simulink model "single_link"  (R2023b)
settings: Solver=VariableStepAuto  StartTime=0.0  StopTime=100  RelTol=1e-3
undefined symbols (not defined in the file): X, Y, Z
libraries: sm_lib x10, nesl_utility x3
settings Model: Creator=Admin  LastModifiedBy=gughan
settings ModelReferenceCC: EnableRefExpFcnMdlSchedulingChecks=on

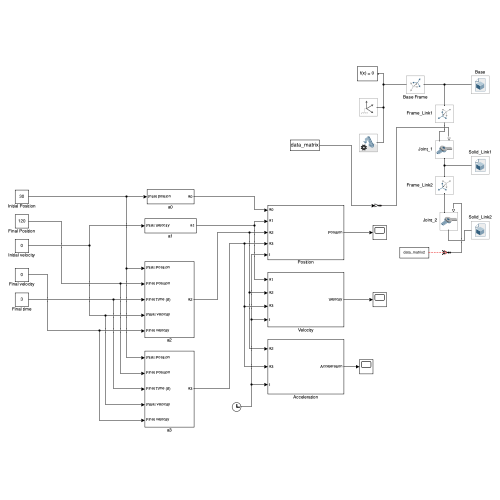
[thumbnail: Simulink's stored preview of the top-level diagram]
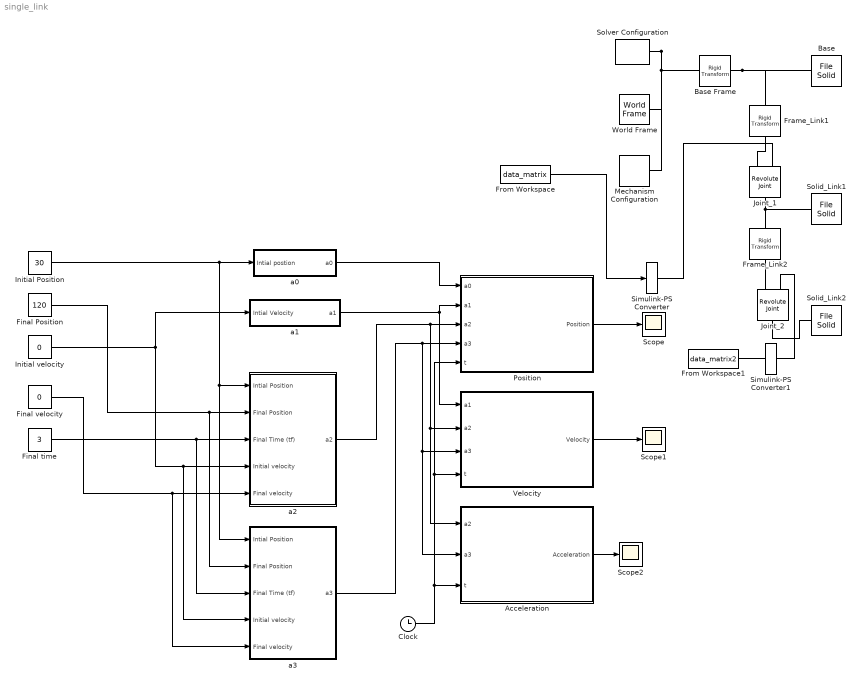
== system single_link ==
  Acceleration : Subsystem
  Base : sm_lib/Body Elements/File Solid  ExtGeomFileName=/Users/gughan/Documents/VIT VELLORE STUFFS/TP/base1.STEP  UnitType=FromFile  ExtGeomFileUnits=m  StepReaderType=HEX  ExportConvexHullGeometry=off  InertiaType=CalculateFromGeometry  Mass=1  MassUnits=kg  CenterOfMass=[0 0 0]  CenterOfMassUnits=m  MomentsOfInertia=[1 1 1]  MomentsOfInertiaUnits=kg*m^2  ProductsOfInertia=[0 0 0]  ProductsOfInertiaUnits=kg*m^2  BasedOnType=Density  Density=1000  DensityUnits=kg/m^3  DoExposeReferenceFrame=on  SerializedFrames=<Frames/>  GraphicType=FromGeometry  MarkerShape=Sphere  MarkerSize=10  GraphicVisPropType=SimpleVisualProperties  GraphicDiffuseColor=[0.5 0.5 0.5]  GraphicSpecularColor=[0.5 0.5 0.5 1.0]  GraphicAmbientColor=[0.15 0.15 0.15 1.0]  GraphicEmissiveColor=[0.0 0.0 0.0 1.0]  GraphicShininess=75  GraphicOpacity=1.0
  Base Frame : sm_lib/Frames and Transforms/Rigid Transform  TranslationMethod=Cartesian  TranslationStandardOffset=0  TranslationStandardOffsetUnits=m  TranslationStandardAxis=+Z  TranslationCartesianOffset=[0 0 0]  TranslationCartesianOffsetUnits=m  TranslationROffset=0  TranslationROffsetUnits=m  TranslationZOffset=0  TranslationZOffsetUnits=m  TranslationThetaOffset=0  TranslationThetaOffsetUnits=deg  RotationMethod=None  RotationAngleUnits=deg  RotationStandardAxis=+X  RotationAngle=90  RotationArbitraryAxis=[0 0 1]  FollAlignAxisA=+X  BaseAlignAxisA=+Y  FollAlignAxisB=+Y  BaseAlignAxisB=+Z  RotationSequenceAxes=FollowerAxes  RotationSequence=XYX  RotationSequenceAngles=[0 0 0]  RotationSequenceAnglesUnits=deg  RotationMatrix=[1 0 0; 0 1 0; 0 0 1]  Quaternion=[1 0 0 0]
  Clock : Clock
      settings: Decimation=3
  Final Position : Constant  Value=120
  Final time : Constant  Value=3
  Final velocity : Constant  Value=0
  Frame_Link1 : sm_lib/Frames and Transforms/Rigid Transform  TranslationMethod=Cartesian  TranslationStandardOffset=0  TranslationStandardOffsetUnits=mm  TranslationStandardAxis=+Z  TranslationCartesianOffset=[0 0 15]  TranslationCartesianOffsetUnits=mm  TranslationROffset=0  TranslationROffsetUnits=m  TranslationZOffset=0  TranslationZOffsetUnits=m  TranslationThetaOffset=0  TranslationThetaOffsetUnits=deg  RotationMethod=None  RotationAngleUnits=deg  RotationStandardAxis=+X  RotationAngle=90  RotationArbitraryAxis=[0 0 1]  FollAlignAxisA=+X  BaseAlignAxisA=+Y  FollAlignAxisB=+Y  BaseAlignAxisB=+Z  RotationSequenceAxes=FollowerAxes  RotationSequence=XYX  RotationSequenceAngles=[0 0 0]  RotationSequenceAnglesUnits=deg  RotationMatrix=[1 0 0; 0 1 0; 0 0 1]  Quaternion=[1 0 0 0]
  Frame_Link2 : sm_lib/Frames and Transforms/Rigid Transform  TranslationMethod=Cartesian  TranslationStandardOffset=0  TranslationStandardOffsetUnits=mm  TranslationStandardAxis=+Z  TranslationCartesianOffset=[200 0 10]  TranslationCartesianOffsetUnits=mm  TranslationROffset=0  TranslationROffsetUnits=m  TranslationZOffset=0  TranslationZOffsetUnits=m  TranslationThetaOffset=0  TranslationThetaOffsetUnits=deg  RotationMethod=None  RotationAngleUnits=deg  RotationStandardAxis=+Z  RotationAngle=0.0  RotationArbitraryAxis=[0 0 1]  FollAlignAxisA=+X  BaseAlignAxisA=+Y  FollAlignAxisB=+Y  BaseAlignAxisB=+Z  RotationSequenceAxes=FollowerAxes  RotationSequence=XYX  RotationSequenceAngles=[0 0 0]  RotationSequenceAnglesUnits=deg  RotationMatrix=[1 0 0; 0 1 0; 0 0 1]  Quaternion=[1 0 0 0]
  From Workspace : FromWorkspace  VariableName=data_matrix
  From Workspace1 : FromWorkspace  VariableName=data_matrix2
  Initial Position : Constant  Value=30
  Initial velocity : Constant  Value=0
  Joint_1 : sm_lib/Joints/Revolute Joint  JointMode=Normal  SenseConstraintForce=off  SenseConstraintForceX=off  SenseConstraintForceY=off  SenseConstraintForceZ=off  SenseConstraintTorque=off  SenseConstraintTorqueX=off  SenseConstraintTorqueY=off  SenseConstraintTorqueZ=off  SenseTotalForce=off  SenseTotalForceX=off  SenseTotalForceY=off  SenseTotalForceZ=off  SenseTotalTorque=off  SenseTotalTorqueX=off  SenseTotalTorqueY=off  SenseTotalTorqueZ=off  CompositeWrenchDir=FollowerOnBase  CompositeWrenchFrame=BaseFrame  EquilibriumPosition=0  EquilibriumPositionUnits=deg  SpringStiffness=0  SpringStiffnessUnits=N*m/deg  DampingCoefficient=0  DampingCoefficientUnits=N*m/(deg/s)  TorqueActuationMode=ComputedTorque  MotionActuationMode=InputMotion  SensePosition=off  SenseVelocity=off  SenseAcceleration=off  SenseTorqueForce=off  SenseLowerLimitTorqueForce=off  SenseUpperLimitTorqueForce=off  LowerLimitSpecify=off  LowerLimitBound=-90  LowerLimitBoundUnits=deg  LowerLimitStiffness=1e4  LowerLimitStiffnessUnits=N*m/deg  LowerLimitDamping=10  LowerLimitDampingUnits=N*m/(deg/s)  LowerLimitTransitionRegionWidth=0.1  LowerLimitTransitionRegionWidthUnits=deg  UpperLimitSpecify=off  UpperLimitBound=90  UpperLimitBoundUnits=deg  UpperLimitStiffness=1e4  UpperLimitStiffnessUnits=N*m/deg  UpperLimitDamping=10  UpperLimitDampingUnits=N*m/(deg/s)  UpperLimitTransitionRegionWidth=0.1  UpperLimitTransitionRegionWidthUnits=deg  PositionTargetSpecify=off  PositionTargetPriority=High  PositionTargetValue=0  PositionTargetValueUnits=deg  VelocityTargetSpecify=off  VelocityTargetPriority=High  VelocityTargetValue=0  VelocityTargetValueUnits=deg/s
  Joint_2 : sm_lib/Joints/Revolute Joint  JointMode=Normal  SenseConstraintForce=off  SenseConstraintForceX=off  SenseConstraintForceY=off  SenseConstraintForceZ=off  SenseConstraintTorque=off  SenseConstraintTorqueX=off  SenseConstraintTorqueY=off  SenseConstraintTorqueZ=off  SenseTotalForce=off  SenseTotalForceX=off  SenseTotalForceY=off  SenseTotalForceZ=off  SenseTotalTorque=off  SenseTotalTorqueX=off  SenseTotalTorqueY=off  SenseTotalTorqueZ=off  CompositeWrenchDir=FollowerOnBase  CompositeWrenchFrame=BaseFrame  EquilibriumPosition=0  EquilibriumPositionUnits=deg  SpringStiffness=0  SpringStiffnessUnits=N*m/deg  DampingCoefficient=0  DampingCoefficientUnits=N*m/(deg/s)  TorqueActuationMode=ComputedTorque  MotionActuationMode=InputMotion  SensePosition=off  SenseVelocity=off  SenseAcceleration=off  SenseTorqueForce=off  SenseLowerLimitTorqueForce=off  SenseUpperLimitTorqueForce=off  LowerLimitSpecify=off  LowerLimitBound=-90  LowerLimitBoundUnits=deg  LowerLimitStiffness=1e4  LowerLimitStiffnessUnits=N*m/deg  LowerLimitDamping=10  LowerLimitDampingUnits=N*m/(deg/s)  LowerLimitTransitionRegionWidth=0.1  LowerLimitTransitionRegionWidthUnits=deg  UpperLimitSpecify=off  UpperLimitBound=90  UpperLimitBoundUnits=deg  UpperLimitStiffness=1e4  UpperLimitStiffnessUnits=N*m/deg  UpperLimitDamping=10  UpperLimitDampingUnits=N*m/(deg/s)  UpperLimitTransitionRegionWidth=0.1  UpperLimitTransitionRegionWidthUnits=deg  PositionTargetSpecify=off  PositionTargetPriority=High  PositionTargetValue=0  PositionTargetValueUnits=deg  VelocityTargetSpecify=off  VelocityTargetPriority=High  VelocityTargetValue=0  VelocityTargetValueUnits=deg/s
  Mechanism Configuration : sm_lib/Utilities/Mechanism Configuration  UniformGravity=Constant  GravityVector=[0 0 -9.80665]  GravityVectorUnits=m/s^2  LinearizationDelta=0.001  JointModeTransitionNonlinearIterations=2
  Position : Subsystem
  Scope : Scope
  Scope1 : Scope
  Scope2 : Scope
  Simulink-PS Converter : nesl_utility/Simulink-PS Converter  PhysicalDomain=network_engine_domain  SubClassName=ps_input  LeftPortType=input  RightPortType=output  PseudoPeriodic=off  Frequencies=[]  NoiseDistribution=none  NoiseParameters=[]  Unit=deg  AffineConversion=off  FilteringAndDerivatives=filter  SimscapeFilterOrder=2  InputFilterTimeConstant=.01  UdotUserProvided=0
  Simulink-PS Converter1 : nesl_utility/Simulink-PS Converter  PhysicalDomain=network_engine_domain  SubClassName=ps_input  LeftPortType=input  RightPortType=output  PseudoPeriodic=off  Frequencies=[]  NoiseDistribution=none  NoiseParameters=[]  Unit=deg  AffineConversion=off  FilteringAndDerivatives=filter  SimscapeFilterOrder=2  InputFilterTimeConstant=.01  UdotUserProvided=0
  Solid_Link1 : sm_lib/Body Elements/File Solid  ExtGeomFileName=/Users/gughan/Documents/VIT VELLORE STUFFS/TP/link1.STEP  UnitType=FromFile  ExtGeomFileUnits=m  StepReaderType=HEX  ExportConvexHullGeometry=off  InertiaType=CalculateFromGeometry  Mass=1  MassUnits=kg  CenterOfMass=[0 0 0]  CenterOfMassUnits=m  MomentsOfInertia=[1 1 1]  MomentsOfInertiaUnits=kg*m^2  ProductsOfInertia=[0 0 0]  ProductsOfInertiaUnits=kg*m^2  BasedOnType=Density  Density=1000  DensityUnits=kg/m^3  DoExposeReferenceFrame=on  SerializedFrames=<Frames/>  GraphicType=FromGeometry  MarkerShape=Sphere  MarkerSize=10  GraphicVisPropType=SimpleVisualProperties  GraphicDiffuseColor=[0.5 0.5 0.5]  GraphicSpecularColor=[0.5 0.5 0.5 1.0]  GraphicAmbientColor=[0.15 0.15 0.15 1.0]  GraphicEmissiveColor=[0.0 0.0 0.0 1.0]  GraphicShininess=75  GraphicOpacity=1.0
  Solid_Link2 : sm_lib/Body Elements/File Solid  ExtGeomFileName=/Users/gughan/Documents/VIT VELLORE STUFFS/TP/link1.STEP  UnitType=FromFile  ExtGeomFileUnits=m  StepReaderType=HEX  ExportConvexHullGeometry=off  InertiaType=CalculateFromGeometry  Mass=1  MassUnits=kg  CenterOfMass=[0 0 0]  CenterOfMassUnits=m  MomentsOfInertia=[1 1 1]  MomentsOfInertiaUnits=kg*m^2  ProductsOfInertia=[0 0 0]  ProductsOfInertiaUnits=kg*m^2  BasedOnType=Density  Density=1000  DensityUnits=kg/m^3  DoExposeReferenceFrame=on  SerializedFrames=<Frames/>  GraphicType=FromGeometry  MarkerShape=Sphere  MarkerSize=10  GraphicVisPropType=SimpleVisualProperties  GraphicDiffuseColor=[0.5 0.5 0.5]  GraphicSpecularColor=[0.5 0.5 0.5 1.0]  GraphicAmbientColor=[0.15 0.15 0.15 1.0]  GraphicEmissiveColor=[0.0 0.0 0.0 1.0]  GraphicShininess=75  GraphicOpacity=1.0
  Solver Configuration : nesl_utility/Solver Configuration  PhysicalDomain=network_engine_domain  SubClassName=solver  LeftPortType=input  RightPortType=generic  Tones=[]  Harmonics=[]  SimulateNoise=off  Profile=off  UseLocalSampling=off  EnableSwitchedLinearOptims=on  FrequencyDomain=off  UseCCode=off  RelTol=0.001  AbsTol=1e-06  MinStep=1e-09  ToWorkspace=off  RevertToSquareIcSolve=off  NumHomotopyIterations=100  PhasorMode=off  PhasorModeNumHarmonics=1  ConsistencySolver=NEWTON_FTOL  IndexReductionMethod=DerivativeReplacement  DoDC=off  ResidualTolerance=1e-09  ConsistencyTolSource=GLOBAL  ConsistencyAbsTol=0.001  ConsistencyRelTol=0.001  ConsistencyTolFactor=0.001  UseLocalSolver=off  LocalSolverChoice=NE_BACKWARD_EULER_ADVANCER  ResolveIndetEquations=on  FunctionEvalNumThread=1  LocalSolverSampleTime=0.001  DoFixedCost=off  MaxNonlinIter=3  MaxModeIter=2  ComputeImpulses=off  ImpulseIterations=2  LinearAlgebra=auto  LinearAlgebraNumThread=0  EquationFormulation=NE_TIME_EF  DelaysMemoryBudget=1024  AutomaticFiltering=on  FilteringTimeConstant=0.001  PartitionStorageMethod=AS_NEEDED  PartitionMemoryBudget=1024  PartitionMethod=ROBUST  MultibodyUseLocalSolver=off  MultibodyLocalSolverChoice=ODE1  MultibodyLocalSolverSampleTime=0.001
  Velocity : Subsystem
  World Frame : sm_lib/Frames and Transforms/World Frame
  a0 : Subsystem
  a1 : Subsystem
  a2 : Subsystem
  a3 : Subsystem
  wires:
  Acceleration/1(Acceleration) -> Scope2/1
  Velocity/1(Velocity) -> Scope1/1
  Clock/1 -> Velocity/4(t), Position/5(t), Acceleration/3(t)
  a3/1(a3) -> Acceleration/2(a3), Velocity/3(a3), Position/4(a3)
  Initial Position/1 -> a3/1("Intial Position "), a2/1("Intial Position "), a0/1("Intial postion ")
  a0/1(a0) -> Position/1(a0)
  Initial velocity/1 -> a3/4(Initial velocity), a2/4(Initial velocity), a1/1("Intial Velocity ")
  Final velocity/1 -> a3/5(Final velocity), a2/5(Final velocity)
  Final time/1 -> a3/3(Final Time (tf)), a2/3(Final Time (tf))
  Position/1(Position) -> Scope/1
  Final Position/1 -> a3/2(Final Position), a2/2(Final Position)
  a1/1(a1) -> Velocity/1(a1), Position/2(a1)
  a2/1(a2) -> Acceleration/1(a2), Velocity/2(a2), Position/3(a2)
  From Workspace/1 -> Simulink-PS Converter/1
  From Workspace1/1 -> ?
  connections:
  Base Frame/RConn1 -- Base/RConn1 -- Frame_Link1/LConn1
  Joint_1/RConn1 -- Frame_Link2/LConn1 -- Solid_Link1/RConn1
  Solver Configuration/RConn1 -- Mechanism Configuration/RConn1 -- World Frame/RConn1 -- Base Frame/LConn1
  Joint_1/LConn1 -- Frame_Link1/RConn1
  Joint_2/LConn1 -- Frame_Link2/RConn1
  Solid_Link2/RConn1 -- Joint_2/RConn1
  Simulink-PS Converter1/RConn1 -- Joint_2/LConn2
  Joint_1/LConn2 -- Simulink-PS Converter/RConn1

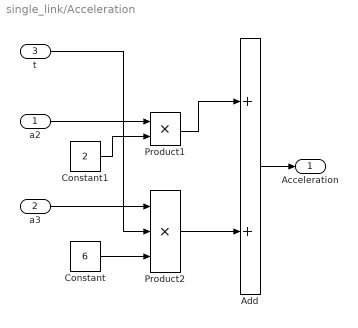
== system single_link/Acceleration ==
  a2 : Inport
  a3 : Inport  Port=2
  t : Inport  Port=3
  Add : Sum
  Constant : Constant  Value=6
  Constant1 : Constant  Value=2
  Product1 : Product
  Product2 : Product  Inputs=3
  Acceleration : Outport
  wires:
  a3/1 -> Product2/1
  t/1 -> Product2/2
  a2/1 -> Product1/1
  Add/1 -> Acceleration/1
  Product2/1 -> Add/2
  Constant/1 -> Product2/3
  Constant1/1 -> Product1/2
  Product1/1 -> Add/1

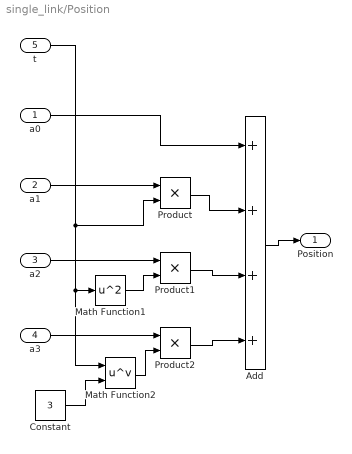
== system single_link/Position ==
  a0 : Inport
  a1 : Inport  Port=2
  a2 : Inport  Port=3
  a3 : Inport  Port=4
  t : Inport  Port=5
  Add : Sum  Inputs=++++
  Constant : Constant  Value=3
  Math Function1 : Math  Operator=square
  Math Function2 : Math  Operator=pow
  Product : Product
  Product1 : Product
  Product2 : Product
  Position : Outport
  wires:
  a1/1 -> Product/1
  Constant/1 -> Math Function2/2
  Math Function1/1 -> Product1/2
  a3/1 -> Product2/1
  Product1/1 -> Add/3
  t/1 -> Product/2, Math Function1/1, Math Function2/1
  Math Function2/1 -> Product2/2
  a2/1 -> Product1/1
  Product2/1 -> Add/4
  Add/1 -> Position/1
  Product/1 -> Add/2
  a0/1 -> Add/1

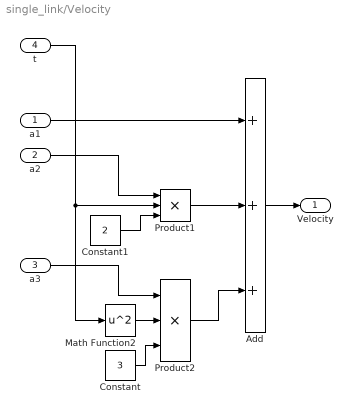
== system single_link/Velocity ==
  a1 : Inport
  a2 : Inport  Port=2
  a3 : Inport  Port=3
  t : Inport  Port=4
  Add : Sum  Inputs=+++
  Constant : Constant  Value=3
  Constant1 : Constant  Value=2
  Math Function2 : Math  Operator=square
  Product1 : Product  Inputs=3
  Product2 : Product  Inputs=3
  Velocity : Outport
  wires:
  a1/1 -> Add/1
  t/1 -> Math Function2/1, Product1/2
  a3/1 -> Product2/1
  Math Function2/1 -> Product2/2
  a2/1 -> Product1/1
  Add/1 -> Velocity/1
  Product1/1 -> Add/2
  Constant1/1 -> Product1/3
  Product2/1 -> Add/3
  Constant/1 -> Product2/3

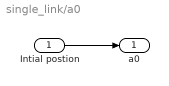
== system single_link/a0 ==
  "Intial postion " : Inport
  a0 : Outport
  wires:
  "Intial postion "/1 -> a0/1

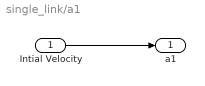
== system single_link/a1 ==
  "Intial Velocity " : Inport
  a1 : Outport
  wires:
  "Intial Velocity "/1 -> a1/1

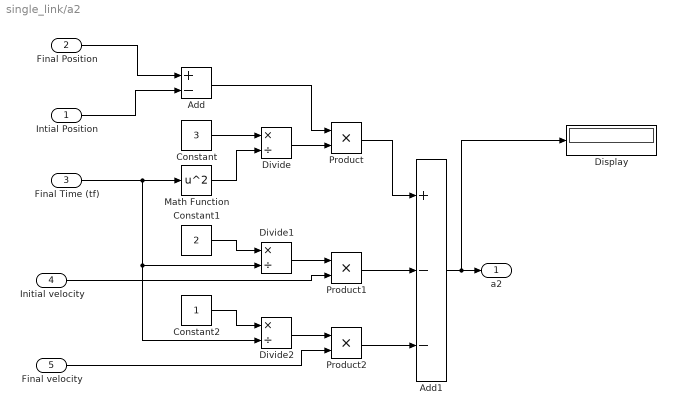
== system single_link/a2 ==
  "Intial Position " : Inport
  Final Position : Inport  Port=2
  Final Time (tf) : Inport  Port=3
  Initial velocity : Inport  Port=4
  Final velocity : Inport  Port=5
  Add : Sum  Inputs=+-
  Add1 : Sum  Inputs=+--
  Constant : Constant  Value=3
  Constant1 : Constant  Value=2
  Constant2 : Constant
  Display : Display
  Divide : Product  Inputs=*/
  Divide1 : Product  Inputs=*/
  Divide2 : Product  Inputs=*/
  Math Function : Math  Operator=square
  Product : Product
  Product1 : Product
  Product2 : Product
  a2 : Outport
  wires:
  Final Time (tf)/1 -> Divide2/2, Divide1/2, Math Function/1
  Constant/1 -> Divide/1
  Math Function/1 -> Divide/2
  "Intial Position "/1 -> Add/2
  Final Position/1 -> Add/1
  Divide/1 -> Product/2
  Add/1 -> Product/1
  Constant1/1 -> Divide1/1
  Divide1/1 -> Product1/1
  Initial velocity/1 -> Product1/2
  Constant2/1 -> Divide2/1
  Final velocity/1 -> Product2/2
  Divide2/1 -> Product2/1
  Add1/1 -> Display/1, a2/1
  Product/1 -> Add1/1
  Product1/1 -> Add1/2
  Product2/1 -> Add1/3

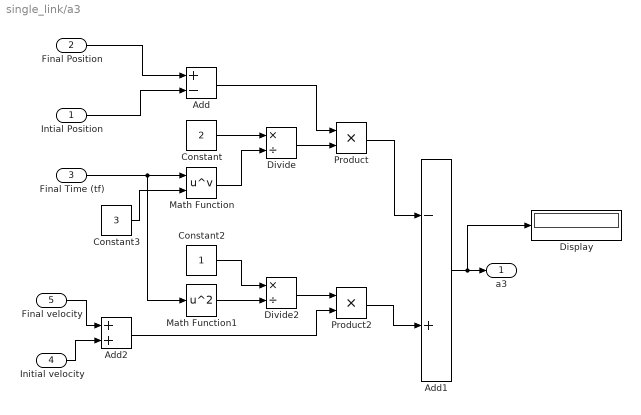
== system single_link/a3 ==
  "Intial Position " : Inport
  Final Position : Inport  Port=2
  Final Time (tf) : Inport  Port=3
  Initial velocity : Inport  Port=4
  Final velocity : Inport  Port=5
  Add : Sum  Inputs=+-
  Add1 : Sum  Inputs=-+
  Add2 : Sum
  Constant : Constant  Value=2
  Constant2 : Constant
  Constant3 : Constant  Value=3
  Display : Display
  Divide : Product  Inputs=*/
  Divide2 : Product  Inputs=*/
  Math Function : Math  Operator=pow
  Math Function1 : Math  Operator=square
  Product : Product
  Product2 : Product
  a3 : Outport
  wires:
  Final Time (tf)/1 -> Math Function1/1, Math Function/1
  Constant/1 -> Divide/1
  Math Function/1 -> Divide/2
  "Intial Position "/1 -> Add/2
  Final Position/1 -> Add/1
  Divide/1 -> Product/2
  Add/1 -> Product/1
  Constant2/1 -> Divide2/1
  Divide2/1 -> Product2/1
  Add1/1 -> Display/1, a3/1
  Product/1 -> Add1/1
  Product2/1 -> Add1/2
  Constant3/1 -> Math Function/2
  Math Function1/1 -> Divide2/2
  Final velocity/1 -> Add2/1
  Initial velocity/1 -> Add2/2
  Add2/1 -> Product2/2
